simulink model "Q3sim5"  (R2022a)
settings: Solver=VariableStepAuto  StartTime=0.0  StopTime=60  FixedStep=1e-4  RelTol=1e-6
values from neighbouring files (symbols this model uses):
  Am = M    (= 0)    [Q3.m]
  Bm = N    (= 1)    [Q3.m]
  C = [1 0 0 0]    [Q3.m]
  K = Ka (1:4)    [Q3.m]
  Km = Ka(5)    [Q3.m]
settings Model: Creator=Crippa  LastModifiedBy=Crippa
settings SolverCC: ZeroCrossControl=DisableAll

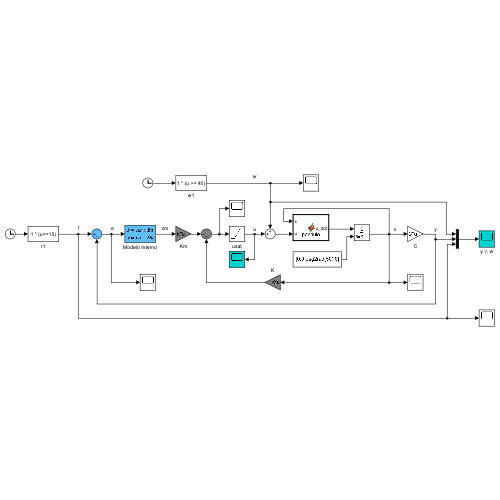
[thumbnail: Simulink's stored preview of the top-level diagram]
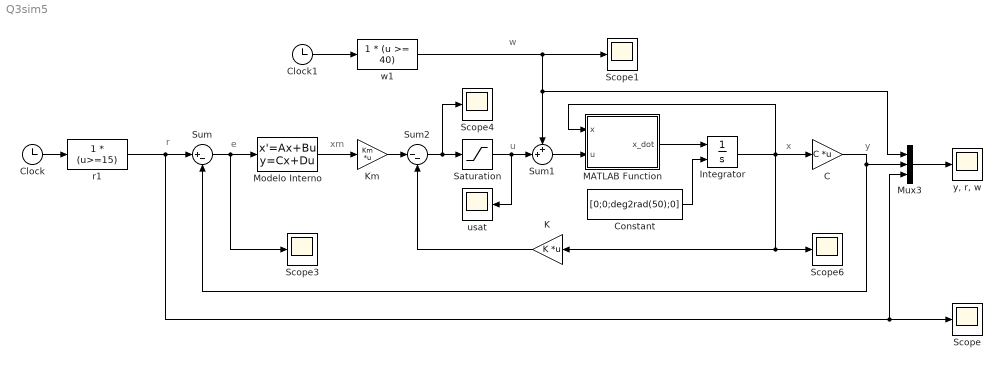
== system Q3sim5 ==
  note: xm
  note: r
  note: x
  note: u
  note: e
  note: y
  note: w
  C : Gain  Gain=C  Multiplication=Matrix(K*u)
  Clock : Clock
  Clock1 : Clock
  Constant : Constant  Value=[0;0;deg2rad(50);0]  VectorParams1D=off
  Integrator : Integrator  InitialConditionSource=external
  K : Gain  Gain=K  Multiplication=Matrix(K*u)
  Km : Gain  Gain=Km  Multiplication=Matrix(K*u)
  MATLAB Function : MATLAB Function  TreatAsAtomicUnit=on
  Modelo Interno : StateSpace  A=Am  B=Bm  C=eye(1)  D=zeros(1)  InitialCondition=0
  Mux3 : Mux  Inputs=3
  Saturation : Saturate  UpperLimit=150  LowerLimit=-150
  Scope{,1,3..4,6} (5 alike) : Scope
  Sum : Sum  Inputs=|+-
  Sum1 : Sum  Inputs=++|
  Sum2 : Sum  Inputs=|--
  r1 : Fcn  Expr=1 * (u>=15)
  usat : Scope
  w1 : Fcn  Expr=1 * (u >= 40)
  "y, r, w" : Scope
  wires:
  K/1 -> Sum2/2
  Modelo Interno/1 -> Km/1
  r1/1 -> Sum/1, Scope/1, Mux3/3
  Km/1 -> Sum2/1
  Sum2/1 -> Saturation/1, Scope4/1
  Clock/1 -> r1/1
  Mux3/1 -> "y, r, w"/1
  Sum/1 -> Modelo Interno/1, Scope3/1
  C/1 -> Mux3/2, Sum/2
  Saturation/1 -> Sum1/2, usat/1
  Clock1/1 -> w1/1
  w1/1 -> Scope1/1, Mux3/1, Sum1/1
  Sum1/1 -> MATLAB Function/2(u)
  MATLAB Function/1(x_dot) -> Integrator/1
  Integrator/1 -> MATLAB Function/1(x), C/1, Scope6/1, K/1
  Constant/1 -> Integrator/2

== matlab function Q3sim5/MATLAB Function ==
  data: x input; u input; x_dot output
function x_dot = pendulo(x,u)
    % x1 = y, x2 = y', x3 = theta, x4 = theta'

    % Parâmetros do pêndulo invertido
    M = 1; 
    m = 0.5;
    L = 1; 
    g = 9.81;

    x1 = x(1);
    x2 = x(2);
    x3 = x(3);
    x4 = x(4);

    % Dinâmica dos estados
    f1 = x2;
    f2 = (-m*g*sin(x3)*cos(x3) + m*L*(x4^2)*sin(x3)) / (M+m-m*cos(x3)^2);
    f3 = x4;
    f4 = g*sin(x3)/L - f2*cos(x3)/L;
    
    % Dinâmica do controle
    g1 = 0;
    g2 = u/(M+m-m*cos(x3)^2);
    g3 = 0;
    g4 = -cos(x3)/L * u/(M+m-m*cos(x3)^2);
    
    f = [f1; f2; f3; f4];
    g = [g1; g2; g3; g4];

    x_dot = f + g;
end
